simulink model "controllerB1_10nodes_test"  (R2021b)
settings: Solver=ode8  StartTime=0.0  StopTime=5  FixedStep=0.001  MaxStep=.1  RelTol=1e-3
settings Model: Creator=imi  LastModifiedBy=ASUS
settings SolverCC: AlgebraicLoopSolver=TrustRegion
settings DataIOCC: SaveFormat=StructureWithTime  ReturnWorkspaceOutputs=off
settings OptimizationCC: LifeSpan=inf
settings DebuggingCC: SFExecutionAtInitializationDiag=none  SFMachineParentedDataDiag=warning  ArithmeticOperatorsInVariantConditions=warning
settings HardwareCC: ProdBitPerSizeT=32  ProdBitPerPtrDiffT=32  ProdWordSize=32  ProdHWDeviceType=Specified
settings SFSimCC: SimUseLocalCustomCode=off  CustomCodeUndefinedFunction=UseInterfaceOnly
settings RTWCC: RTWUseLocalCustomCode=off
settings CodeAppCC: StateflowObjectComments=on

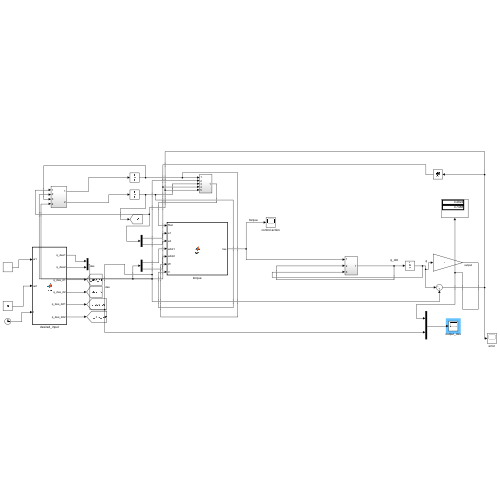
[thumbnail: Simulink's stored preview of the top-level diagram]
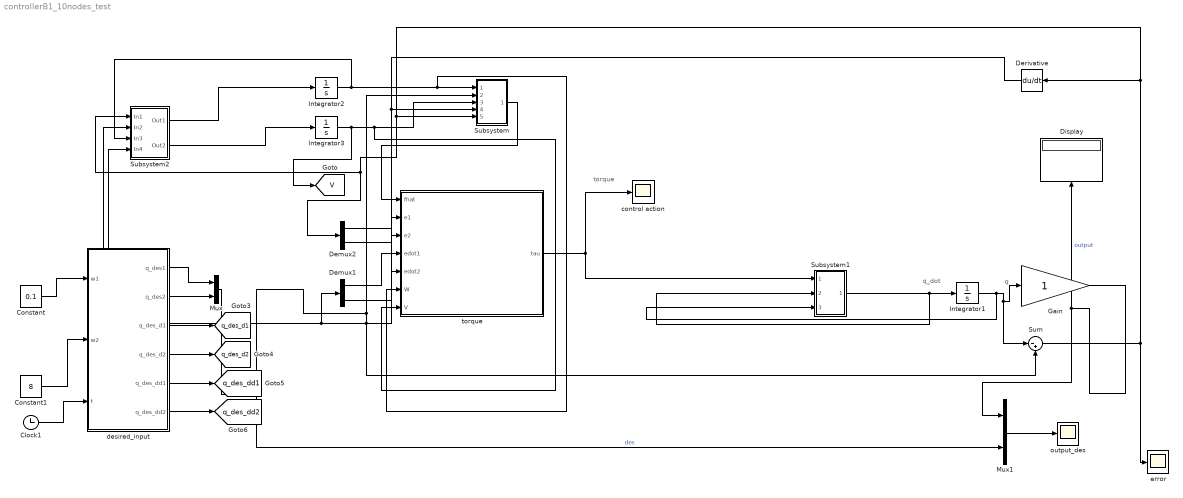
== system controllerB1_10nodes_test ==
  note: torque
  note: q
  note: q_dot
  Clock1 : Clock
  Constant : Constant  Value=0.1
  Constant1 : Constant  Value=8
  Demux1 : Demux  Outputs=2
  Demux2 : Demux  Outputs=2
  Derivative : Derivative
  Display : Display
  Gain : Gain
  Integrator1 : Integrator  InitialCondition=[45;95]*pi/180*0
  Integrator2 : Integrator  InitialCondition=zeros(2,10)
  Integrator3 : Integrator  InitialCondition=zeros(10,11)
  Mux : Mux  Inputs=2
  Mux1 : Mux  Inputs=2
  Subsystem : Subsystem
  Subsystem1 : Subsystem
  Subsystem2 : Subsystem
  Sum : Sum  Inputs=|-+
  control action : Scope
  desired_input : MATLAB Function  TreatAsAtomicUnit=on
  error : Scope
  output_des : Scope
  torque : MATLAB Function  TreatAsAtomicUnit=on
  tag scope: V=global, q_des_d1=global, q_des_d2=global, q_des_dd1=global, q_des_dd2=global
  wires:
  Integrator1/1 -> Subsystem1/3(In3), Sum/1, Gain/1
  torque/1(tau) -> Subsystem1/1(In1), control action/1
  Gain/1 -> Mux1/1, Display/1  "output"
  Mux/1 -> Mux1/2, Subsystem/2(In2), Subsystem2/4(In4), Sum/2  "des"
  Integrator2/1 -> Subsystem2/3(In3), torque/6(W), Subsystem/1(In1)
  Integrator3/1 -> [V], Subsystem/3(In3), torque/7(V)
  Derivative/1 -> Demux1/1, Subsystem2/2(In2), Subsystem/4(In4)
  Sum/1 -> error/1, Derivative/1, Demux2/1, Subsystem2/1(In1), Subsystem/5(In5)
  Subsystem1/1(Out1) -> Subsystem1/2(In2), Integrator1/1
  Subsystem2/1(Out1) -> Integrator2/1
  Subsystem2/2(Out2) -> Integrator3/1
  Subsystem/1(Out1) -> torque/1(fhat)
  Demux2/1 -> torque/2(e1)
  Demux2/2 -> torque/3(e2)
  Demux1/1 -> torque/4(edot1)
  Demux1/2 -> torque/5(edot2)
  desired_input/1(q_des1) -> Mux/1
  desired_input/2(q_des2) -> Mux/2
  Mux1/1 -> output_des/1
  Clock1/1 -> desired_input/3(t)
  Constant1/1 -> desired_input/2(w2)
  Constant/1 -> desired_input/1(w1)
  desired_input/3(q_des_d1) -> [q_des_d1]
  desired_input/4(q_des_d2) -> [q_des_d2]
  desired_input/5(q_des_dd1) -> [q_des_dd1]
  desired_input/6(q_des_dd2) -> [q_des_dd2]

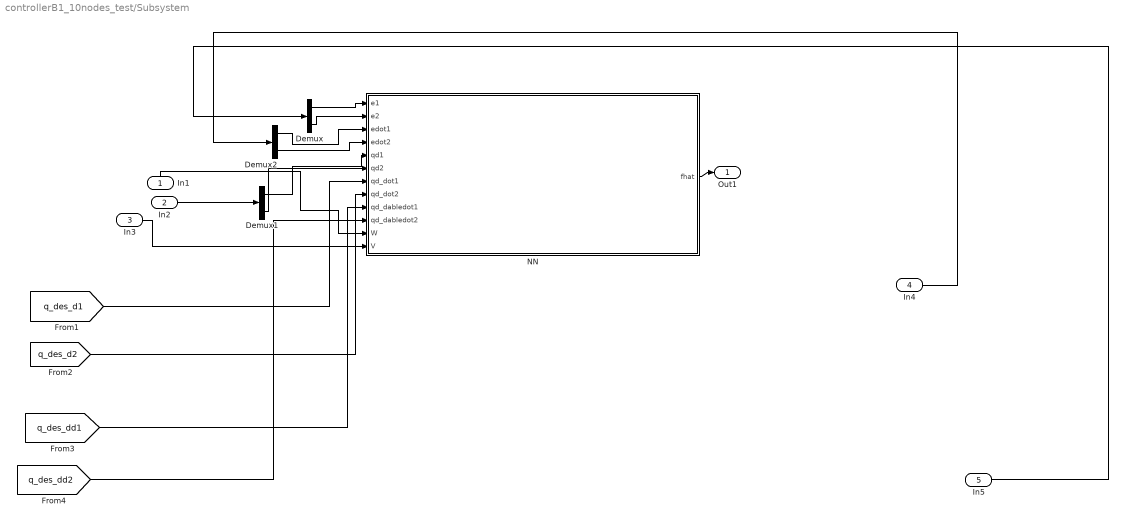
== system controllerB1_10nodes_test/Subsystem ==
  In1 : Inport
  In2 : Inport  Port=2
  In3 : Inport  Port=3
  In4 : Inport  Port=4
  In5 : Inport  Port=5
  Demux : Demux  Outputs=2
  Demux1 : Demux  Outputs=2
  Demux2 : Demux  Outputs=2
  NN : MATLAB Function  TreatAsAtomicUnit=on
  Out1 : Outport
  wires:
  Demux2/1 -> NN/3(edot1)
  In4/1 -> Demux2/1
  [q_des_d2] -> NN/8(qd_dot2)
  Demux/2 -> NN/2(e2)
  In5/1 -> Demux/1
  Demux1/2 -> NN/6(qd2)
  Demux/1 -> NN/1(e1)
  [q_des_d1] -> NN/7(qd_dot1)
  Demux1/1 -> NN/5(qd1)
  [q_des_dd2] -> NN/10(qd_dabledot2)
  [q_des_dd1] -> NN/9(qd_dabledot1)
  Demux2/2 -> NN/4(edot2)
  NN/1(fhat) -> Out1/1
  In1/1 -> NN/11(W)
  In2/1 -> Demux1/1
  In3/1 -> NN/12(V)

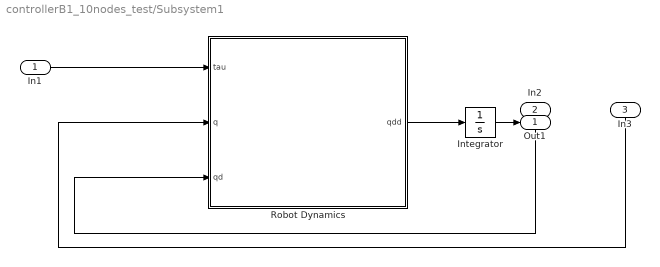
== system controllerB1_10nodes_test/Subsystem1 ==
  In1 : Inport
  In2 : Inport  Port=2
  In3 : Inport  Port=3
  Integrator : Integrator  InitialCondition=zeros(2,1)
  Robot Dynamics : MATLAB Function  TreatAsAtomicUnit=on
  Out1 : Outport
  wires:
  Robot Dynamics/1(qdd) -> Integrator/1
  Integrator/1 -> Out1/1
  In3/1 -> Robot Dynamics/2(q)
  In2/1 -> Robot Dynamics/3(qd)
  In1/1 -> Robot Dynamics/1(tau)

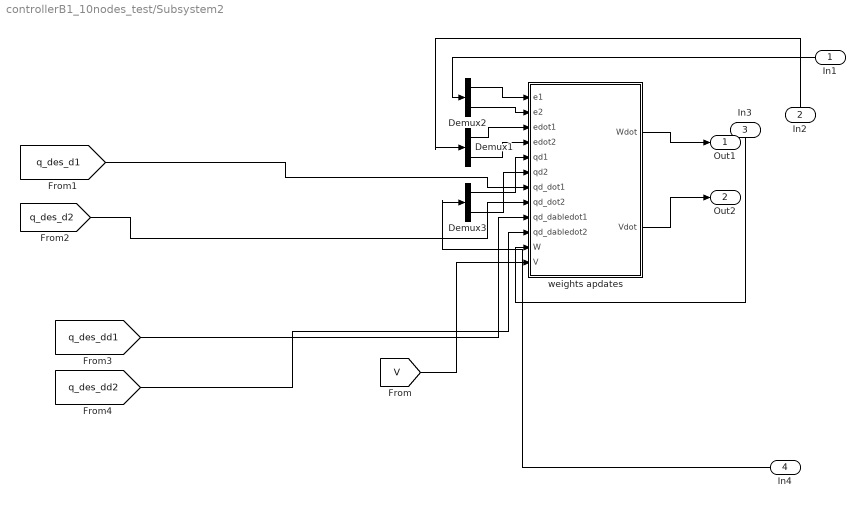
== system controllerB1_10nodes_test/Subsystem2 ==
  In1 : Inport
  In2 : Inport  Port=2
  In3 : Inport  Port=3
  In4 : Inport  Port=4
  Demux1 : Demux  Outputs=2
  Demux2 : Demux  Outputs=2
  Demux3 : Demux  Outputs=2
  weights apdates : MATLAB Function  TreatAsAtomicUnit=on
  Out1 : Outport
  Out2 : Outport  Port=2
  wires:
  [q_des_d1] -> weights apdates/7(qd_dot1)
  [q_des_d2] -> weights apdates/8(qd_dot2)
  weights apdates/1(Wdot) -> Out1/1
  Demux1/2 -> weights apdates/4(edot2)
  Demux1/1 -> weights apdates/3(edot1)
  weights apdates/2(Vdot) -> Out2/1
  Demux2/2 -> weights apdates/2(e2)
  Demux3/1 -> weights apdates/5(qd1)
  In2/1 -> Demux1/1
  In4/1 -> Demux3/1
  In1/1 -> Demux2/1
  In3/1 -> weights apdates/11(W)
  Demux2/1 -> weights apdates/1(e1)
  Demux3/2 -> weights apdates/6(qd2)
  [V] -> weights apdates/12(V)
  [q_des_dd1] -> weights apdates/9(qd_dabledot1)
  [q_des_dd2] -> weights apdates/10(qd_dabledot2)

== matlab function controllerB1_10nodes_test/torque ==
  data: fhat input; e1 input; tau output; e2 input; edot1 input; edot2 input; W input; V input
function tau = fcn(fhat,e1,e2,edot1,edot2,W,V)
e = [e1 e2];
edot = [edot1 edot2];
%filtered error:
r = edot' + 10*eye(2)*e';

Z = [V W']; 
%design constants:
Kv = 20;
Kz = 1;
% ZM = norm(Z,'fro');
ZM = sqrt((2*80*(1.62e-05)^2)+(80*11*(1.458e-05)^2));
v = -Kz*((norm(Z,'fro'))+ZM)*r;
tau = fhat + Kv*r - v;

== matlab function controllerB1_10nodes_test/Subsystem1/Robot Dynamics ==
  data: tau input; q input; qdd output; qd input
function qdd = fcn(tau,q,qd)

q1=q(1);
q2=q(2);

q1d=qd(1);
q2d=qd(2);



m1=.1;
m2=.1;

I1=.01;
I2=.01;

l1=.12;
l2=.1;

lc1=l1/2;
lc2=l2/2;


g=9.8;



d11=m1*lc1^2+m2*(l1^2+lc2^2+2*l1*lc2^2+2*l1*l2*cos(q2))+I1+I2;
d12=m2*(lc2^2+l1*l2*cos(q2))+I2;
d22=m2*lc2^2+I2;

h=-m2*l1*lc2*sin(q2);

c121=h;
c211=h;
c112=-h;
c221=h;



M=[d11,d12;d12,d22];
C=[c121*q2d,c211*q1d+c221*q2d;c112*q1d,0];
G=[(m1*lc1+m2*l1)*g*cos(q1)+m2*lc2*g*cos(q1+q2);m2*lc2*cos(q1+q2)];


qdd=pinv(M)*((tau)-C*qd-G*0);

== matlab function controllerB1_10nodes_test/Subsystem/NN ==
  data: e1 input; fhat output; e2 input; edot1 input; edot2 input; qd1 input; qd2 input; qd_dot1 input; qd_dot2 input; qd_dabledot1 input; qd_dabledot2 input; W input; V input
function fhat = NNcontroller(e1,e2,edot1,edot2,qd1,qd2,qd_dot1,qd_dot2,qd_dabledot1,qd_dabledot2,W,V)
% inputs: 5*3
e = [e1 e2];
edot = [edot1 edot2];
qd = [qd1 qd2];
qd_dot = [qd_dot1 qd_dot2];
qd_dabledot = [qd_dabledot1 qd_dabledot2];
X = transpose([e edot qd qd_dot qd_dabledot 1]);
% X: 11*1 &  W:2*10 &  V:10*11  
%input:11  & hidden:10  &  output:2


%%forward
A = zeros(10,1);
A = V*X;
for i = 1:10    
     A(i,1) = sigmoid(A(i,1));    
end

fhat = W*A;

== matlab function controllerB1_10nodes_test/Subsystem2/weights apdates ==
  data: e1 input; e2 input; edot1 input; edot2 input; qd1 input; qd2 input; qd_dot1 input; qd_dot2 input; qd_dabledot1 input; qd_dabledot2 input; Wdot output; W input; Vdot output; V input
function [Wdot,Vdot] = fcn(e1,e2,edot1,edot2,qd1,qd2,qd_dot1,qd_dot2,qd_dabledot1,qd_dabledot2,W,V)
% e = [e1;e2];
% edot = [edot1;edot2];
% qd = [qd1;qd2];
% qd_dot = [qd_dot1;qd_dot2];
% qd_dabledot = [qd_dabledot1;qd_dabledot2];
% X = [e' ; edot' ; qd' ; qd_dot' ; qd_dabledot'];
e = [e1 e2];
edot = [edot1 edot2];
qd = [qd1 qd2];
qd_dot = [qd_dot1 qd_dot2];
qd_dabledot = [qd_dabledot1 qd_dabledot2];
X = transpose([e edot qd qd_dot qd_dabledot 1]);

%filtered error:
r = edot' + 10*eye(2)*e';
% if r(1,1)>=0.5
%     r(1,1)=0.5;
% elseif r(1,1)<=-0.5
%     r(1,1)=-0.5;
% end
% 
% if r(2,1)>=0.5
%     r(2,1)=0.5;
% elseif r(2,1)<=-0.5
%     r(2,1)=-0.5;
% end

r_sig = [0;0];
r_sig(1,1) = sigmoid(r(1,1));
r_sig(2,1) = sigmoid(r(2,1));

G = ones(11,11);
F = ones(10,10);
k = 2;
rr = zeros(10,2);
rr(1,1) = r_sig(1,1);
rr(1,2) = r_sig(2,1);



Wdot_T = F*rr - (F*V*X*r') - (k*F*norm(r)*W');
Vdot_T = G*X*(transpose(W'*r)) - (k*G*norm(r)*V');


% Wdot_T = F * r_sig';
% Vdot_T = G * X * temp1;
Wdot = Wdot_T';
Vdot = Vdot_T';
end

== matlab function controllerB1_10nodes_test/desired_input ==
  data: w1 input; q_des1 output; w2 input; q_des2 output; q_des_d1 output; q_des_d2 output; q_des_dd1 output; q_des_dd2 output; t input
function [q_des1,q_des2,q_des_d1,q_des_d2,q_des_dd1,q_des_dd2] = fcn(w1,w2,t)
q_des1 = sin(w1*t);
q_des2 = sin(w2*t);

q_des_d1 = w1*(cos(w1*t));
q_des_d2 = w2*(cos(w2*t));

q_des_dd1 = -w1^2*(sin(w1*t));
q_des_dd2 = -w2^2*(sin(w2*t));
